simulink library "MESSIN_Library"  (R2024a)
settings: Solver=VariableStepAuto  StartTime=0.0  StopTime=10.0  RelTol=1e-3
undefined symbols (not defined in the file or in its folder): actuatorCommand, commandedActuator, commandMode, externCommand, ready, remoteControlDevice, sensor, supervisor, timestampUTC, useXNAllocation
libraries: $bdroot x376, etargetslib x52, simulink x19
(part 4 of 5)

== system MESSIN_Library/State Message/Unpack MESSIN State Message/unpack message/Unpack AirMAR ==
  busIn : Inport
  bytes : Inport  Port=2
  Bus Assignment : BusAssignment  AssignedSignals=sensor.airMAR.air.timestampUTC,sensor.airMAR.air.pressure,sensor.airMAR.air.airTemperature,sensor.airMAR.relativeWind.timestampUTC,sensor.airMAR.relativeWind.windAngle,sensor.airMAR.relativeWind.windSpeed
  Byte Unpack : etargetslib/Byte Unpack  dimensions={1,1,1,1,1,1}  datatypes={'double','single','single','double','single','single'}  byteAlign=1
      settings: LibrarySourceBlock=embeddedtargetslib/Host Communication/Byte Unpack
  Convert Double Network Byte Order : $bdroot/Utilities/Convert Double Network Byte Order
  Convert Double Network Byte Order1 : $bdroot/Utilities/Convert Double Network Byte Order
  Convert Single Network Byte Order{,1..3} (4 alike) : $bdroot/Utilities/Convert Single Network Byte Order
  Data Type Conversion{1..2,9..12} (6 alike) : DataTypeConversion  OutDataTypeStr=double  SaturateOnIntegerOverflow=off  RndMeth=Floor
  Signal Specification1 : SignalSpecification  OutDataTypeStr=double  Unit=s  Dimensions=1
  Signal Specification12 : SignalSpecification  OutDataTypeStr=double  Unit=s  Dimensions=1
  Signal Specification17 : SignalSpecification  OutDataTypeStr=double  Unit=rad  Dimensions=1
  Signal Specification18 : SignalSpecification  OutDataTypeStr=double  Unit=m/s  Dimensions=1
  Signal Specification2 : SignalSpecification  OutDataTypeStr=double  Unit=Pa  Dimensions=1
  Signal Specification3 : SignalSpecification  OutDataTypeStr=double  Unit=°C  Dimensions=1
  busOut : Outport
  wires:
  Bus Assignment/1 -> busOut/1
  bytes/1 -> Byte Unpack/1
  busIn/1 -> Bus Assignment/1
  Byte Unpack/1 -> Convert Double Network Byte Order/1
  Byte Unpack/2 -> Convert Single Network Byte Order/1
  Byte Unpack/3 -> Convert Single Network Byte Order1/1
  Data Type Conversion9/1 -> Signal Specification1/1
  Data Type Conversion10/1 -> Signal Specification2/1
  Data Type Conversion11/1 -> Signal Specification3/1
  Data Type Conversion12/1 -> Signal Specification12/1
  Data Type Conversion2/1 -> Signal Specification18/1
  Data Type Conversion1/1 -> Signal Specification17/1
  Signal Specification1/1 -> Bus Assignment/2  "timestampUTC"
  Signal Specification12/1 -> Bus Assignment/5  "timestampUTC"
  Signal Specification17/1 -> Bus Assignment/6  "windAngle"
  Signal Specification2/1 -> Bus Assignment/3  "pressure"
  Signal Specification18/1 -> Bus Assignment/7  "windSpeed"
  Signal Specification3/1 -> Bus Assignment/4  "airTemperature"
  Convert Double Network Byte Order/1 -> Data Type Conversion9/1
  Convert Single Network Byte Order/1 -> Data Type Conversion10/1
  Convert Single Network Byte Order1/1 -> Data Type Conversion11/1
  Byte Unpack/4 -> Convert Double Network Byte Order1/1
  Byte Unpack/5 -> Convert Single Network Byte Order2/1
  Byte Unpack/6 -> Convert Single Network Byte Order3/1
  Convert Double Network Byte Order1/1 -> Data Type Conversion12/1
  Convert Single Network Byte Order2/1 -> Data Type Conversion1/1
  Convert Single Network Byte Order3/1 -> Data Type Conversion2/1

== system MESSIN_Library/State Message/Unpack MESSIN State Message/unpack message/Unpack AllocationCommand ==
  busIn : Inport
  bytes : Inport  Port=2
  Bus Assignment : BusAssignment  AssignedSignals=externCommand.allocationCommand.XYN
  Byte Unpack : etargetslib/Byte Unpack  dimensions={1,1,1}  datatypes={'double','double','double'}  byteAlign=1
      settings: LibrarySourceBlock=embeddedtargetslib/Host Communication/Byte Unpack
  Convert Double Network Byte Order : $bdroot/Utilities/Convert Double Network Byte Order
  Convert Double Network Byte Order1 : $bdroot/Utilities/Convert Double Network Byte Order
  Convert Double Network Byte Order2 : $bdroot/Utilities/Convert Double Network Byte Order
  Make Finite : $bdroot/Utilities/Make Finite
  Make Finite1 : $bdroot/Utilities/Make Finite
  Make Finite2 : $bdroot/Utilities/Make Finite
  Mux : Mux  Inputs=3
  Signal Specification1 : SignalSpecification  OutDataTypeStr=double  Dimensions=3
  busOut : Outport
  wires:
  Byte Unpack/3 -> Convert Double Network Byte Order2/1
  Byte Unpack/2 -> Convert Double Network Byte Order1/1
  Byte Unpack/1 -> Convert Double Network Byte Order/1
  Convert Double Network Byte Order2/1 -> Make Finite2/1
  Convert Double Network Byte Order1/1 -> Make Finite1/1
  Convert Double Network Byte Order/1 -> Make Finite/1
  Bus Assignment/1 -> busOut/1
  bytes/1 -> Byte Unpack/1
  busIn/1 -> Bus Assignment/1
  Signal Specification1/1 -> Bus Assignment/2  "XYN"
  Make Finite2/1 -> Mux/3
  Make Finite1/1 -> Mux/2
  Make Finite/1 -> Mux/1
  Mux/1 -> Signal Specification1/1

== system MESSIN_Library/State Message/Unpack MESSIN State Message/unpack message/Unpack BMS ==
  busIn : Inport
  bytes : Inport  Port=2
  Bus Assignment : BusAssignment  AssignedSignals=sensor.batteryManagementSystem.batteryStarboard.timestampUTC,sensor.batteryManagementSystem.batteryStarboard.voltage,sensor.batteryManagementSystem.batteryStarboard.current,sensor.batteryManagementSystem.batteryStarboard.consumedElectricCharge,sensor.batteryManagementSystem.batteryStarboard.stateOfCharge,sensor.batteryManagementSystem.batteryPortside.timestampUTC,sensor.batteryManagementSystem.batteryPortside.voltage,sensor.batteryManagementSystem.batteryPortside.current,sensor.batteryManagementSystem.batteryPortside.consumedElectricCharge,sensor.batteryManagementSystem.batteryPortside.stateOfCharge
  Byte Unpack : etargetslib/Byte Unpack  dimensions={1,1,1,1,1,1,1,1,1,1}  datatypes={'double','single','single','single','single','double','single','single','single','single'}  byteAlign=1
      settings: LibrarySourceBlock=embeddedtargetslib/Host Communication/Byte Unpack
  Convert Double Network Byte Order : $bdroot/Utilities/Convert Double Network Byte Order
  Convert Double Network Byte Order2 : $bdroot/Utilities/Convert Double Network Byte Order
  Convert Single Network Byte Order{,1..7} (8 alike) : $bdroot/Utilities/Convert Single Network Byte Order
  Data Type Conversion{1..3,5..11} (10 alike) : DataTypeConversion  OutDataTypeStr=double  SaturateOnIntegerOverflow=off  RndMeth=Floor
  Signal Specification17 : SignalSpecification  OutDataTypeStr=double  Unit=A*s  Dimensions=1
  Signal Specification18 : SignalSpecification  OutDataTypeStr=double  Unit=1  Dimensions=1
  Signal Specification19 : SignalSpecification  OutDataTypeStr=double  Unit=A*s  Dimensions=1
  Signal Specification20 : SignalSpecification  OutDataTypeStr=double  Unit=1  Dimensions=1
  Signal Specification21 : SignalSpecification  OutDataTypeStr=double  Unit=s  Dimensions=1
  Signal Specification22 : SignalSpecification  OutDataTypeStr=double  Unit=V  Dimensions=1
  Signal Specification23 : SignalSpecification  OutDataTypeStr=double  Unit=A  Dimensions=1
  Signal Specification24 : SignalSpecification  OutDataTypeStr=double  Unit=s  Dimensions=1
  Signal Specification25 : SignalSpecification  OutDataTypeStr=double  Unit=V  Dimensions=1
  Signal Specification26 : SignalSpecification  OutDataTypeStr=double  Unit=A  Dimensions=1
  busOut : Outport
  wires:
  busIn/1 -> Bus Assignment/1
  bytes/1 -> Byte Unpack/1
  Bus Assignment/1 -> busOut/1
  Convert Double Network Byte Order/1 -> Data Type Conversion5/1
  Convert Single Network Byte Order/1 -> Data Type Conversion6/1
  Convert Single Network Byte Order1/1 -> Data Type Conversion7/1
  Convert Single Network Byte Order2/1 -> Data Type Conversion8/1
  Convert Double Network Byte Order2/1 -> Data Type Conversion10/1
  Convert Single Network Byte Order4/1 -> Data Type Conversion11/1
  Convert Single Network Byte Order3/1 -> Data Type Conversion9/1
  Data Type Conversion5/1 -> Signal Specification24/1
  Data Type Conversion6/1 -> Signal Specification25/1
  Data Type Conversion7/1 -> Signal Specification26/1
  Data Type Conversion8/1 -> Signal Specification17/1
  Data Type Conversion9/1 -> Signal Specification18/1
  Data Type Conversion10/1 -> Signal Specification21/1
  Data Type Conversion11/1 -> Signal Specification22/1
  Signal Specification24/1 -> Bus Assignment/2  "timestampUTC"
  Signal Specification19/1 -> Bus Assignment/10  "consumedElectricCharge"
  Signal Specification20/1 -> Bus Assignment/11  "stateOfCharge"
  Signal Specification25/1 -> Bus Assignment/3  "voltage"
  Signal Specification26/1 -> Bus Assignment/4  "current"
  Signal Specification21/1 -> Bus Assignment/7  "timestampUTC"
  Signal Specification17/1 -> Bus Assignment/5  "consumedElectricCharge"
  Signal Specification22/1 -> Bus Assignment/8  "voltage"
  Signal Specification23/1 -> Bus Assignment/9  "current"
  Signal Specification18/1 -> Bus Assignment/6  "stateOfCharge"
  Data Type Conversion2/1 -> Signal Specification20/1
  Data Type Conversion1/1 -> Signal Specification19/1
  Data Type Conversion3/1 -> Signal Specification23/1
  Convert Single Network Byte Order7/1 -> Data Type Conversion3/1
  Convert Single Network Byte Order6/1 -> Data Type Conversion2/1
  Convert Single Network Byte Order5/1 -> Data Type Conversion1/1
  Byte Unpack/1 -> Convert Double Network Byte Order/1
  Byte Unpack/2 -> Convert Single Network Byte Order/1
  Byte Unpack/3 -> Convert Single Network Byte Order1/1
  Byte Unpack/4 -> Convert Single Network Byte Order2/1
  Byte Unpack/5 -> Convert Single Network Byte Order3/1
  Byte Unpack/6 -> Convert Double Network Byte Order2/1
  Byte Unpack/7 -> Convert Single Network Byte Order4/1
  Byte Unpack/8 -> Convert Single Network Byte Order7/1
  Byte Unpack/9 -> Convert Single Network Byte Order5/1
  Byte Unpack/10 -> Convert Single Network Byte Order6/1

== system MESSIN_Library/State Message/Unpack MESSIN State Message/unpack message/Unpack CommandedActuator ==
  busIn : Inport
  bytes : Inport  Port=2
  Bus Assignment : BusAssignment  AssignedSignals=commandedActuator.throttleStarboard,commandedActuator.throttlePortside,commandedActuator.angleStarboard,commandedActuator.anglePortside
  Byte Unpack : etargetslib/Byte Unpack  dimensions={1,1,1,1}  datatypes={'double','double','double','double'}  byteAlign=1
      settings: LibrarySourceBlock=embeddedtargetslib/Host Communication/Byte Unpack
  Convert Double Network Byte Order{,1..3} (4 alike) : $bdroot/Utilities/Convert Double Network Byte Order
  Data Type Conversion{5..8} (4 alike) : DataTypeConversion  OutDataTypeStr=double  SaturateOnIntegerOverflow=off  RndMeth=Floor
  Make Finite{,1..3} (4 alike) : $bdroot/Utilities/Make Finite
  Signal Specification1 : SignalSpecification  OutDataTypeStr=double  Unit=1  Dimensions=1
  Signal Specification2 : SignalSpecification  OutDataTypeStr=double  Unit=1  Dimensions=1
  Signal Specification3 : SignalSpecification  OutDataTypeStr=double  Unit=rad  Dimensions=1
  Signal Specification4 : SignalSpecification  OutDataTypeStr=double  Unit=rad  Dimensions=1
  busOut : Outport
  wires:
  Byte Unpack/4 -> Convert Double Network Byte Order3/1
  Byte Unpack/3 -> Convert Double Network Byte Order2/1
  Byte Unpack/2 -> Convert Double Network Byte Order1/1
  Byte Unpack/1 -> Convert Double Network Byte Order/1
  Make Finite3/1 -> Signal Specification4/1
  Make Finite2/1 -> Signal Specification3/1
  Make Finite1/1 -> Signal Specification1/1
  Data Type Conversion6/1 -> Make Finite1/1
  Make Finite/1 -> Signal Specification2/1
  Convert Double Network Byte Order3/1 -> Data Type Conversion8/1
  Convert Double Network Byte Order2/1 -> Data Type Conversion7/1
  Convert Double Network Byte Order1/1 -> Data Type Conversion6/1
  Convert Double Network Byte Order/1 -> Data Type Conversion5/1
  Data Type Conversion8/1 -> Make Finite3/1
  Data Type Conversion7/1 -> Make Finite2/1
  Data Type Conversion5/1 -> Make Finite/1
  Bus Assignment/1 -> busOut/1
  bytes/1 -> Byte Unpack/1
  busIn/1 -> Bus Assignment/1
  Signal Specification4/1 -> Bus Assignment/5  "anglePortside"
  Signal Specification3/1 -> Bus Assignment/4  "angleStarboard"
  Signal Specification1/1 -> Bus Assignment/3  "throttlePortside"
  Signal Specification2/1 -> Bus Assignment/2  "throttleStarboard"

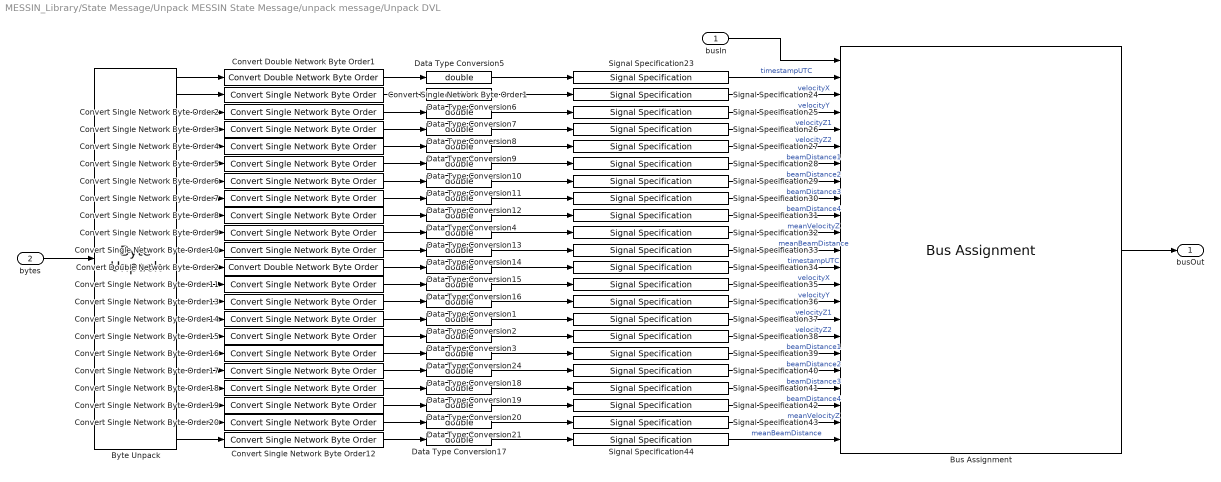
== system MESSIN_Library/State Message/Unpack MESSIN State Message/unpack message/Unpack DVL ==
  busIn : Inport
  bytes : Inport  Port=2
  Bus Assignment : BusAssignment  AssignedSignals=sensor.nortekDVL1000.bottomTrack.timestampUTC,sensor.nortekDVL1000.bottomTrack.velocityX,sensor.nortekDVL1000.bottomTrack.velocityY,sensor.nortekDVL1000.bottomTrack.velocityZ1,sensor.nortekDVL1000.bottomTrack.velocityZ2,sensor.nortekDVL1000.bottomTrack.beamDistance1,sensor.nortekDVL1000.bottomTrack.beamDistance2,sensor.nortekDVL1000.bottomTrack.beamDistance3,sensor.nortekDVL1000.bottomTrack.beamDistance4,sensor.nortekDVL1000.bottomTrack.meanVelocityZ,sensor.nortekDVL1000.bottomTrack.meanBeamDistance,sensor.nortekDVL1000.waterTrack.timestampUTC,sensor.nortekDVL1000.waterTrack.velocityX,sensor.nortekDVL1000.waterTrack.velocityY,sensor.nortekDVL1000.waterTrack.velocityZ1,sensor.nortekDVL1000.waterTrack.velocityZ2,sensor.nortekDVL1000.waterTrack.beamDistance1,sensor.nortekDVL1000.waterTrack.beamDistance2,sensor.nortekDVL1000.waterTrack.beamDistance3,sensor.nortekDVL1000.waterTrack.beamDistance4,sensor.nortekDVL1000.waterTrack.meanVelocityZ,sensor.nortekDVL1000.waterTrack.meanBeamDistance
  Byte Unpack : etargetslib/Byte Unpack  dimensions={1,1,1,1,1,1,1,1,1,1,1,1,1,1,1,1,1,1,1,1,1,1}  datatypes={'double','single','single','single','single','single','single','single','single','single','single','double','single','single','single','single','single','single','single','single','single','single'}  byteAlign=1
      settings: LibrarySourceBlock=embeddedtargetslib/Host Communication/Byte Unpack
  Convert Double Network Byte Order1 : $bdroot/Utilities/Convert Double Network Byte Order
  Convert Double Network Byte Order2 : $bdroot/Utilities/Convert Double Network Byte Order
  Convert Single Network Byte Order{1..20} (20 alike) : $bdroot/Utilities/Convert Single Network Byte Order
  Data Type Conversion{1..21,24} (22 alike) : DataTypeConversion  OutDataTypeStr=double  SaturateOnIntegerOverflow=off  RndMeth=Floor
  Signal Specification23 : SignalSpecification  OutDataTypeStr=double  Unit=s  Dimensions=1
  Signal Specification{24..27,32,35..38,43} (10 alike) : SignalSpecification  OutDataTypeStr=double  Unit=m/s  Dimensions=1
  Signal Specification{28..31,33,39..42,44} (10 alike) : SignalSpecification  OutDataTypeStr=double  Unit=m  Dimensions=1
  Signal Specification34 : SignalSpecification  OutDataTypeStr=double  Unit=s  Dimensions=1
  busOut : Outport
  wires:
  Bus Assignment/1 -> busOut/1
  bytes/1 -> Byte Unpack/1
  busIn/1 -> Bus Assignment/1
  Signal Specification28/1 -> Bus Assignment/7  "beamDistance1"
  Signal Specification31/1 -> Bus Assignment/10  "beamDistance4"
  Signal Specification38/1 -> Bus Assignment/17  "velocityZ2"
  Signal Specification39/1 -> Bus Assignment/18  "beamDistance1"
  Signal Specification30/1 -> Bus Assignment/9  "beamDistance3"
  Signal Specification33/1 -> Bus Assignment/12  "meanBeamDistance"
  Signal Specification41/1 -> Bus Assignment/20  "beamDistance3"
  Signal Specification34/1 -> Bus Assignment/13  "timestampUTC"
  Signal Specification29/1 -> Bus Assignment/8  "beamDistance2"
  Signal Specification42/1 -> Bus Assignment/21  "beamDistance4"
  Signal Specification44/1 -> Bus Assignment/23  "meanBeamDistance"
  Signal Specification25/1 -> Bus Assignment/4  "velocityY"
  Signal Specification26/1 -> Bus Assignment/5  "velocityZ1"
  Signal Specification43/1 -> Bus Assignment/22  "meanVelocityZ"
  Signal Specification36/1 -> Bus Assignment/15  "velocityY"
  Signal Specification32/1 -> Bus Assignment/11  "meanVelocityZ"
  Signal Specification27/1 -> Bus Assignment/6  "velocityZ2"
  Signal Specification23/1 -> Bus Assignment/2  "timestampUTC"
  Signal Specification24/1 -> Bus Assignment/3  "velocityX"
  Signal Specification37/1 -> Bus Assignment/16  "velocityZ1"
  Signal Specification35/1 -> Bus Assignment/14  "velocityX"
  Signal Specification40/1 -> Bus Assignment/19  "beamDistance2"
  Data Type Conversion5/1 -> Signal Specification23/1
  Data Type Conversion6/1 -> Signal Specification24/1
  Data Type Conversion7/1 -> Signal Specification25/1
  Data Type Conversion8/1 -> Signal Specification26/1
  Data Type Conversion9/1 -> Signal Specification27/1
  Data Type Conversion10/1 -> Signal Specification28/1
  Data Type Conversion11/1 -> Signal Specification29/1
  Data Type Conversion12/1 -> Signal Specification30/1
  Data Type Conversion3/1 -> Signal Specification38/1
  Data Type Conversion2/1 -> Signal Specification37/1
  Data Type Conversion1/1 -> Signal Specification36/1
  Data Type Conversion16/1 -> Signal Specification35/1
  Data Type Conversion15/1 -> Signal Specification34/1
  Data Type Conversion14/1 -> Signal Specification33/1
  Data Type Conversion13/1 -> Signal Specification32/1
  Data Type Conversion4/1 -> Signal Specification31/1
  Data Type Conversion24/1 -> Signal Specification39/1
  Data Type Conversion18/1 -> Signal Specification40/1
  Data Type Conversion19/1 -> Signal Specification41/1
  Data Type Conversion20/1 -> Signal Specification42/1
  Data Type Conversion21/1 -> Signal Specification43/1
  Data Type Conversion17/1 -> Signal Specification44/1
  Convert Double Network Byte Order1/1 -> Data Type Conversion5/1
  Convert Single Network Byte Order1/1 -> Data Type Conversion6/1
  Convert Single Network Byte Order2/1 -> Data Type Conversion7/1
  Convert Single Network Byte Order3/1 -> Data Type Conversion8/1
  Convert Single Network Byte Order4/1 -> Data Type Conversion9/1
  Convert Single Network Byte Order5/1 -> Data Type Conversion10/1
  Convert Single Network Byte Order6/1 -> Data Type Conversion11/1
  Convert Single Network Byte Order9/1 -> Data Type Conversion13/1
  Convert Single Network Byte Order8/1 -> Data Type Conversion4/1
  Convert Single Network Byte Order7/1 -> Data Type Conversion12/1
  Convert Single Network Byte Order10/1 -> Data Type Conversion14/1
  Convert Single Network Byte Order12/1 -> Data Type Conversion17/1
  Convert Single Network Byte Order18/1 -> Data Type Conversion19/1
  Convert Single Network Byte Order19/1 -> Data Type Conversion20/1
  Convert Single Network Byte Order20/1 -> Data Type Conversion21/1
  Convert Single Network Byte Order17/1 -> Data Type Conversion18/1
  Convert Single Network Byte Order16/1 -> Data Type Conversion24/1
  Convert Single Network Byte Order15/1 -> Data Type Conversion3/1
  Convert Single Network Byte Order14/1 -> Data Type Conversion2/1
  Convert Single Network Byte Order13/1 -> Data Type Conversion1/1
  Convert Single Network Byte Order11/1 -> Data Type Conversion16/1
  Convert Double Network Byte Order2/1 -> Data Type Conversion15/1
  Byte Unpack/1 -> Convert Double Network Byte Order1/1
  Byte Unpack/2 -> Convert Single Network Byte Order1/1
  Byte Unpack/3 -> Convert Single Network Byte Order2/1
  Byte Unpack/4 -> Convert Single Network Byte Order3/1
  Byte Unpack/5 -> Convert Single Network Byte Order4/1
  Byte Unpack/6 -> Convert Single Network Byte Order5/1
  Byte Unpack/7 -> Convert Single Network Byte Order6/1
  Byte Unpack/8 -> Convert Single Network Byte Order7/1
  Byte Unpack/9 -> Convert Single Network Byte Order8/1
  Byte Unpack/10 -> Convert Single Network Byte Order9/1
  Byte Unpack/11 -> Convert Single Network Byte Order10/1
  Byte Unpack/12 -> Convert Double Network Byte Order2/1
  Byte Unpack/13 -> Convert Single Network Byte Order11/1
  Byte Unpack/14 -> Convert Single Network Byte Order13/1
  Byte Unpack/15 -> Convert Single Network Byte Order14/1
  Byte Unpack/16 -> Convert Single Network Byte Order15/1
  Byte Unpack/17 -> Convert Single Network Byte Order16/1
  Byte Unpack/18 -> Convert Single Network Byte Order17/1
  Byte Unpack/19 -> Convert Single Network Byte Order18/1
  Byte Unpack/20 -> Convert Single Network Byte Order19/1
  Byte Unpack/21 -> Convert Single Network Byte Order20/1
  Byte Unpack/22 -> Convert Single Network Byte Order12/1

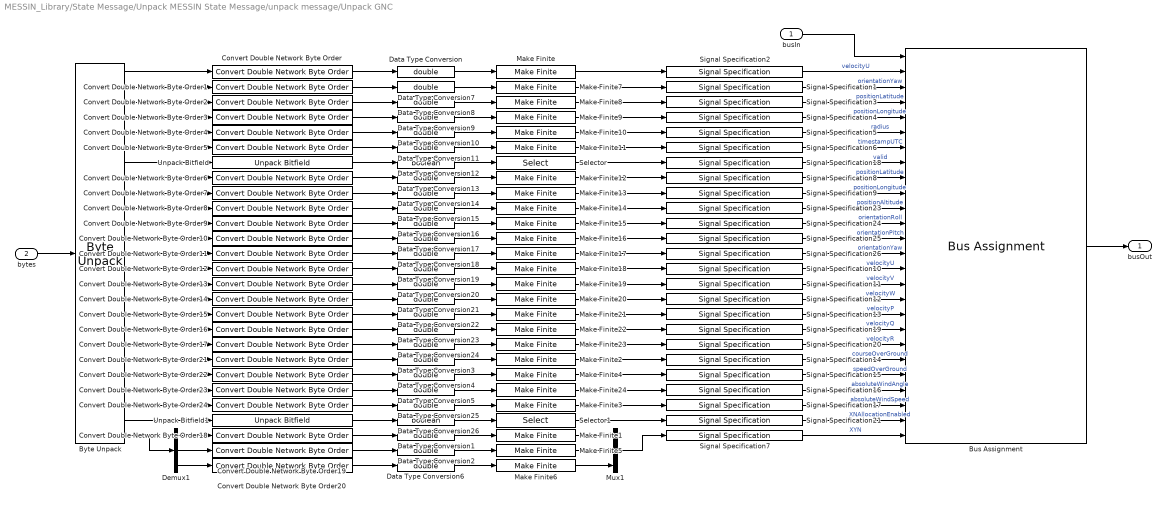
== system MESSIN_Library/State Message/Unpack MESSIN State Message/unpack message/Unpack GNC ==
  busIn : Inport
  bytes : Inport  Port=2
  Bus Assignment : BusAssignment  AssignedSignals=gnc.guidance.surgeHeading.velocityU,gnc.guidance.surgeHeading.orientationYaw,gnc.guidance.stayThere.positionLatitude,gnc.guidance.stayThere.positionLongitude,gnc.guidance.stayThere.radius,gnc.navigation.timestampUTC,gnc.navigation.info.valid,gnc.navigation.state.positionLatitude,gnc.navigation.state.positionLongitude,gnc.navigation.state.positionAltitude,gnc.navigation.state.orientationRoll,gnc.navigation.state.orientationPitch,gnc.navigation.state.orientationYaw,gnc.navigation.state.velocityU,gnc.navigation.state.velocityV,gnc.navigation.state.velocityW,gnc.navigation.state.velocityP,gnc.navigation.state.velocityQ,gnc.navigation.state.velocityR,gnc.navigation.state.courseOverGround,gnc.navigation.state.speedOverGround,gnc.navigation.state.absoluteWindAngle,gnc.navigation.state.absoluteWindSpeed,gnc.control.XNAllocationEnabled,gnc.control.XYN
  Byte Unpack : etargetslib/Byte Unpack  dimensions={1,1,1,1,1,1,1,1,1,1,1,1,1,1,1,1,1,1,1,1,1,1,1,1,3}  datatypes={'double','double','double','double','double','double','uint8','double','double','double','double','double','double','double','double','double','double','double','double','double','double','double','double','uint8','double'}  byteAlign=1
      settings: LibrarySourceBlock=embeddedtargetslib/Host Communication/Byte Unpack
  Convert Double Network Byte Order{,1..24} (25 alike) : $bdroot/Utilities/Convert Double Network Byte Order
  Data Type Conversion{,1..11,13..25} (25 alike) : DataTypeConversion  OutDataTypeStr=double  SaturateOnIntegerOverflow=off  RndMeth=Floor
  Data Type Conversion12 : DataTypeConversion  OutDataTypeStr=boolean  SaturateOnIntegerOverflow=off  RndMeth=Floor
  Data Type Conversion26 : DataTypeConversion  OutDataTypeStr=boolean  SaturateOnIntegerOverflow=off  RndMeth=Floor
  Demux1 : Demux  Outputs=3
  Make Finite{,1..24} (25 alike) : $bdroot/Utilities/Make Finite
  Mux1 : Mux  Inputs=3
  Selector : Selector  InputPortWidth=8  IndexOptions=Index vector (dialog)  Indices=8  OutputSizes=1
  Selector1 : Selector  InputPortWidth=8  IndexOptions=Index vector (dialog)  Indices=8  OutputSizes=1
  Signal Specification{1,3..4,8..9,14,16,24..26} (10 alike) : SignalSpecification  OutDataTypeStr=double  Unit=rad  Dimensions=1
  Signal Specification{2,10..12,15,17} (6 alike) : SignalSpecification  OutDataTypeStr=double  Unit=m/s  Dimensions=1
  Signal Specification13 : SignalSpecification  OutDataTypeStr=double  Unit=rad/s  Dimensions=1
  Signal Specification18 : SignalSpecification  OutDataTypeStr=boolean  Unit=1  Dimensions=1
  Signal Specification19 : SignalSpecification  OutDataTypeStr=double  Unit=rad/s  Dimensions=1
  Signal Specification20 : SignalSpecification  OutDataTypeStr=double  Unit=rad/s  Dimensions=1
  Signal Specification21 : SignalSpecification  OutDataTypeStr=boolean  Unit=1  Dimensions=1
  Signal Specification23 : SignalSpecification  OutDataTypeStr=double  Unit=m  Dimensions=1
  Signal Specification5 : SignalSpecification  OutDataTypeStr=double  Unit=m  Dimensions=1
  Signal Specification6 : SignalSpecification  OutDataTypeStr=double  Unit=s  Dimensions=1
  Signal Specification7 : SignalSpecification  OutDataTypeStr=double  Dimensions=3
  Unpack Bitfield : $bdroot/Utilities/Unpack Bitfield
  Unpack Bitfield1 : $bdroot/Utilities/Unpack Bitfield
  busOut : Outport
  wires:
  Data Type Conversion6/1 -> Make Finite6/1
  Data Type Conversion2/1 -> Make Finite5/1
  Data Type Conversion1/1 -> Make Finite1/1
  Convert Double Network Byte Order18/1 -> Data Type Conversion1/1
  Convert Double Network Byte Order19/1 -> Data Type Conversion2/1
  Convert Double Network Byte Order20/1 -> Data Type Conversion6/1
  Make Finite6/1 -> Mux1/3
  Make Finite5/1 -> Mux1/2
  Make Finite1/1 -> Mux1/1
  Demux1/1 -> Convert Double Network Byte Order18/1
  Demux1/2 -> Convert Double Network Byte Order19/1
  Demux1/3 -> Convert Double Network Byte Order20/1
  Convert Double Network Byte Order/1 -> Data Type Conversion/1
  Data Type Conversion/1 -> Make Finite/1
  busIn/1 -> Bus Assignment/1
  bytes/1 -> Byte Unpack/1
  Bus Assignment/1 -> busOut/1
  Signal Specification3/1 -> Bus Assignment/4  "positionLatitude"
  Signal Specification2/1 -> Bus Assignment/2  "velocityU"
  Signal Specification4/1 -> Bus Assignment/5  "positionLongitude"
  Signal Specification1/1 -> Bus Assignment/3  "orientationYaw"
  Signal Specification5/1 -> Bus Assignment/6  "radius"
  Signal Specification25/1 -> Bus Assignment/13  "orientationPitch"
  Signal Specification23/1 -> Bus Assignment/11  "positionAltitude"
  Signal Specification20/1 -> Bus Assignment/20  "velocityR"
  Signal Specification8/1 -> Bus Assignment/9  "positionLatitude"
  Signal Specification10/1 -> Bus Assignment/15  "velocityU"
  Signal Specification13/1 -> Bus Assignment/18  "velocityP"
  Signal Specification19/1 -> Bus Assignment/19  "velocityQ"
  Signal Specification18/1 -> Bus Assignment/8  "valid"
  Signal Specification11/1 -> Bus Assignment/16  "velocityV"
  Signal Specification6/1 -> Bus Assignment/7  "timestampUTC"
  Signal Specification12/1 -> Bus Assignment/17  "velocityW"
  Signal Specification26/1 -> Bus Assignment/14  "orientationYaw"
  Signal Specification9/1 -> Bus Assignment/10  "positionLongitude"
  Signal Specification24/1 -> Bus Assignment/12  "orientationRoll"
  Signal Specification7/1 -> Bus Assignment/26  "XYN"
  Make Finite/1 -> Signal Specification2/1
  Make Finite7/1 -> Signal Specification1/1
  Data Type Conversion7/1 -> Make Finite7/1
  Convert Double Network Byte Order1/1 -> Data Type Conversion7/1
  Convert Double Network Byte Order3/1 -> Data Type Conversion9/1
  Data Type Conversion9/1 -> Make Finite9/1
  Make Finite9/1 -> Signal Specification4/1
  Make Finite8/1 -> Signal Specification3/1
  Data Type Conversion8/1 -> Make Finite8/1
  Convert Double Network Byte Order2/1 -> Data Type Conversion8/1
  Convert Double Network Byte Order4/1 -> Data Type Conversion10/1
  Data Type Conversion10/1 -> Make Finite10/1
  Make Finite10/1 -> Signal Specification5/1
  Make Finite11/1 -> Signal Specification6/1
  Data Type Conversion11/1 -> Make Finite11/1
  Convert Double Network Byte Order5/1 -> Data Type Conversion11/1
  Data Type Conversion12/1 -> Selector/1
  Unpack Bitfield/1 -> Data Type Conversion12/1
  Selector/1 -> Signal Specification18/1
  Convert Double Network Byte Order8/1 -> Data Type Conversion15/1
  Data Type Conversion15/1 -> Make Finite14/1
  Make Finite14/1 -> Signal Specification23/1
  Make Finite15/1 -> Signal Specification24/1
  Data Type Conversion16/1 -> Make Finite15/1
  Convert Double Network Byte Order9/1 -> Data Type Conversion16/1
  Convert Double Network Byte Order7/1 -> Data Type Conversion14/1
  Data Type Conversion14/1 -> Make Finite13/1
  Make Finite13/1 -> Signal Specification9/1
  Make Finite12/1 -> Signal Specification8/1
  Data Type Conversion13/1 -> Make Finite12/1
  Convert Double Network Byte Order6/1 -> Data Type Conversion13/1
  Convert Double Network Byte Order10/1 -> Data Type Conversion17/1
  Data Type Conversion17/1 -> Make Finite16/1
  Make Finite16/1 -> Signal Specification25/1
  Make Finite17/1 -> Signal Specification26/1
  Data Type Conversion18/1 -> Make Finite17/1
  Convert Double Network Byte Order11/1 -> Data Type Conversion18/1
  Convert Double Network Byte Order13/1 -> Data Type Conversion20/1
  Data Type Conversion20/1 -> Make Finite19/1
  Make Finite19/1 -> Signal Specification11/1
  Make Finite18/1 -> Signal Specification10/1
  Data Type Conversion19/1 -> Make Finite18/1
  Convert Double Network Byte Order12/1 -> Data Type Conversion19/1
  Convert Double Network Byte Order16/1 -> Data Type Conversion23/1
  Data Type Conversion23/1 -> Make Finite22/1
  Make Finite22/1 -> Signal Specification19/1
  Make Finite23/1 -> Signal Specification20/1
  Data Type Conversion24/1 -> Make Finite23/1
  Convert Double Network Byte Order17/1 -> Data Type Conversion24/1
  Convert Double Network Byte Order15/1 -> Data Type Conversion22/1
  Data Type Conversion22/1 -> Make Finite21/1
  Make Finite21/1 -> Signal Specification13/1
  Make Finite20/1 -> Signal Specification12/1
  Data Type Conversion21/1 -> Make Finite20/1
  Convert Double Network Byte Order14/1 -> Data Type Conversion21/1
  Mux1/1 -> Signal Specification7/1
  Byte Unpack/1 -> Convert Double Network Byte Order/1
  Byte Unpack/2 -> Convert Double Network Byte Order1/1
  Byte Unpack/3 -> Convert Double Network Byte Order2/1
  Byte Unpack/4 -> Convert Double Network Byte Order3/1
  Byte Unpack/5 -> Convert Double Network Byte Order4/1
  Byte Unpack/6 -> Convert Double Network Byte Order5/1
  Byte Unpack/7 -> Unpack Bitfield/1
  Byte Unpack/8 -> Convert Double Network Byte Order6/1
  Byte Unpack/9 -> Convert Double Network Byte Order7/1
  Byte Unpack/10 -> Convert Double Network Byte Order8/1
  Byte Unpack/11 -> Convert Double Network Byte Order9/1
  Byte Unpack/12 -> Convert Double Network Byte Order10/1
  Byte Unpack/13 -> Convert Double Network Byte Order11/1
  Byte Unpack/14 -> Convert Double Network Byte Order12/1
  Byte Unpack/15 -> Convert Double Network Byte Order13/1
  Byte Unpack/16 -> Convert Double Network Byte Order14/1
  Byte Unpack/17 -> Convert Double Network Byte Order15/1
  Byte Unpack/18 -> Convert Double Network Byte Order16/1
  Byte Unpack/19 -> Convert Double Network Byte Order17/1
  Convert Double Network Byte Order21/1 -> Data Type Conversion3/1
  Data Type Conversion3/1 -> Make Finite2/1
  Data Type Conversion25/1 -> Make Finite3/1
  Convert Double Network Byte Order24/1 -> Data Type Conversion25/1
  Convert Double Network Byte Order23/1 -> Data Type Conversion5/1
  Data Type Conversion5/1 -> Make Finite24/1
  Data Type Conversion4/1 -> Make Finite4/1
  Convert Double Network Byte Order22/1 -> Data Type Conversion4/1
  Make Finite2/1 -> Signal Specification14/1
  Signal Specification14/1 -> Bus Assignment/21  "courseOverGround"
  Make Finite4/1 -> Signal Specification15/1
  Signal Specification15/1 -> Bus Assignment/22  "speedOverGround"
  Make Finite24/1 -> Signal Specification16/1
  Make Finite3/1 -> Signal Specification17/1
  Signal Specification16/1 -> Bus Assignment/23  "absoluteWindAngle"
  Signal Specification17/1 -> Bus Assignment/24  "absoluteWindSpeed"
  Byte Unpack/20 -> Convert Double Network Byte Order21/1
  Byte Unpack/21 -> Convert Double Network Byte Order22/1
  Byte Unpack/22 -> Convert Double Network Byte Order23/1
  Byte Unpack/23 -> Convert Double Network Byte Order24/1
  Byte Unpack/24 -> Unpack Bitfield1/1
  Unpack Bitfield1/1 -> Data Type Conversion26/1
  Data Type Conversion26/1 -> Selector1/1
  Selector1/1 -> Signal Specification21/1
  Signal Specification21/1 -> Bus Assignment/25  "XNAllocationEnabled"
  Byte Unpack/25 -> Demux1/1

== system MESSIN_Library/State Message/Unpack MESSIN State Message/unpack message/Unpack GNSS ==
  busIn : Inport
  bytes : Inport  Port=2
  Bus Assignment : BusAssignment  AssignedSignals=sensor.gnssAsteRx3.gnss.timestampUTC,sensor.gnssAsteRx3.gnss.latitude,sensor.gnssAsteRx3.gnss.longitude,sensor.gnssAsteRx3.gnss.altitude,sensor.gnssAsteRx3.gnss.hdop,sensor.gnssAsteRx3.gnss.numSat,sensor.gnssAsteRx3.gnss.gpsQuality,sensor.gnssAsteRx3.courseAndSpeedOverGround.timestampUTC,sensor.gnssAsteRx3.courseAndSpeedOverGround.courseOverGround,sensor.gnssAsteRx3.courseAndSpeedOverGround.speedOverGround
  Byte Unpack : etargetslib/Byte Unpack  dimensions={1,1,1,1,1,1,1,1,1,1}  datatypes={'double','double','double','single','single','uint8','uint8','double','single','single'}  byteAlign=1
      settings: LibrarySourceBlock=embeddedtargetslib/Host Communication/Byte Unpack
  Convert Double Network Byte Order{5..8} (4 alike) : $bdroot/Utilities/Convert Double Network Byte Order
  Convert Single Network Byte Order{8..11} (4 alike) : $bdroot/Utilities/Convert Single Network Byte Order
  Data Type Conversion{17,20..21,23..27} (8 alike) : DataTypeConversion  OutDataTypeStr=double  SaturateOnIntegerOverflow=off  RndMeth=Floor
  Data Type Conversion18 : DataTypeConversion  OutDataTypeStr=uint8  SaturateOnIntegerOverflow=off  RndMeth=Floor
  Data Type Conversion19 : DataTypeConversion  OutDataTypeStr=uint8  SaturateOnIntegerOverflow=off  RndMeth=Floor
  Signal Specification45 : SignalSpecification  OutDataTypeStr=double  Unit=m  Dimensions=1
  Signal Specification46 : SignalSpecification  OutDataTypeStr=uint8  Unit=1  Dimensions=1
  Signal Specification47 : SignalSpecification  OutDataTypeStr=double  Unit=m  Dimensions=1
  Signal Specification50 : SignalSpecification  OutDataTypeStr=uint8  Unit=1  Dimensions=1
  Signal Specification51 : SignalSpecification  OutDataTypeStr=double  Unit=s  Dimensions=1
  Signal Specification52 : SignalSpecification  OutDataTypeStr=double  Unit=rad  Dimensions=1
  Signal Specification53 : SignalSpecification  OutDataTypeStr=double  Unit=m/s  Dimensions=1
  Signal Specification54 : SignalSpecification  OutDataTypeStr=double  Unit=s  Dimensions=1
  Signal Specification55 : SignalSpecification  OutDataTypeStr=double  Unit=rad  Dimensions=1
  Signal Specification56 : SignalSpecification  OutDataTypeStr=double  Unit=rad  Dimensions=1
  busOut : Outport
  wires:
  Bus Assignment/1 -> busOut/1
  bytes/1 -> Byte Unpack/1
  busIn/1 -> Bus Assignment/1
  Signal Specification53/1 -> Bus Assignment/11  "speedOverGround"
  Signal Specification46/1 -> Bus Assignment/7  "numSat"
  Signal Specification50/1 -> Bus Assignment/8  "gpsQuality"
  Signal Specification47/1 -> Bus Assignment/6  "hdop"
  Signal Specification55/1 -> Bus Assignment/3  "latitude"
  Signal Specification54/1 -> Bus Assignment/2  "timestampUTC"
  Signal Specification45/1 -> Bus Assignment/5  "altitude"
  Signal Specification52/1 -> Bus Assignment/10  "courseOverGround"
  Signal Specification51/1 -> Bus Assignment/9  "timestampUTC"
  Signal Specification56/1 -> Bus Assignment/4  "longitude"
  Data Type Conversion23/1 -> Signal Specification54/1
  Data Type Conversion24/1 -> Signal Specification55/1
  Data Type Conversion25/1 -> Signal Specification56/1
  Data Type Conversion26/1 -> Signal Specification45/1
  Data Type Conversion27/1 -> Signal Specification47/1
  Data Type Conversion20/1 -> Signal Specification51/1
  Data Type Conversion17/1 -> Signal Specification52/1
  Data Type Conversion21/1 -> Signal Specification53/1
  Data Type Conversion18/1 -> Signal Specification46/1
  Data Type Conversion19/1 -> Signal Specification50/1
  Convert Double Network Byte Order5/1 -> Data Type Conversion23/1
  Convert Double Network Byte Order6/1 -> Data Type Conversion24/1
  Convert Double Network Byte Order7/1 -> Data Type Conversion25/1
  Convert Single Network Byte Order8/1 -> Data Type Conversion26/1
  Convert Single Network Byte Order9/1 -> Data Type Conversion27/1
  Convert Double Network Byte Order8/1 -> Data Type Conversion20/1
  Convert Single Network Byte Order10/1 -> Data Type Conversion17/1
  Convert Single Network Byte Order11/1 -> Data Type Conversion21/1
  Byte Unpack/1 -> Convert Double Network Byte Order5/1
  Byte Unpack/2 -> Convert Double Network Byte Order6/1
  Byte Unpack/3 -> Convert Double Network Byte Order7/1
  Byte Unpack/4 -> Convert Single Network Byte Order8/1
  Byte Unpack/5 -> Convert Single Network Byte Order9/1
  Byte Unpack/6 -> Data Type Conversion18/1
  Byte Unpack/7 -> Data Type Conversion19/1
  Byte Unpack/8 -> Convert Double Network Byte Order8/1
  Byte Unpack/9 -> Convert Single Network Byte Order10/1
  Byte Unpack/10 -> Convert Single Network Byte Order11/1

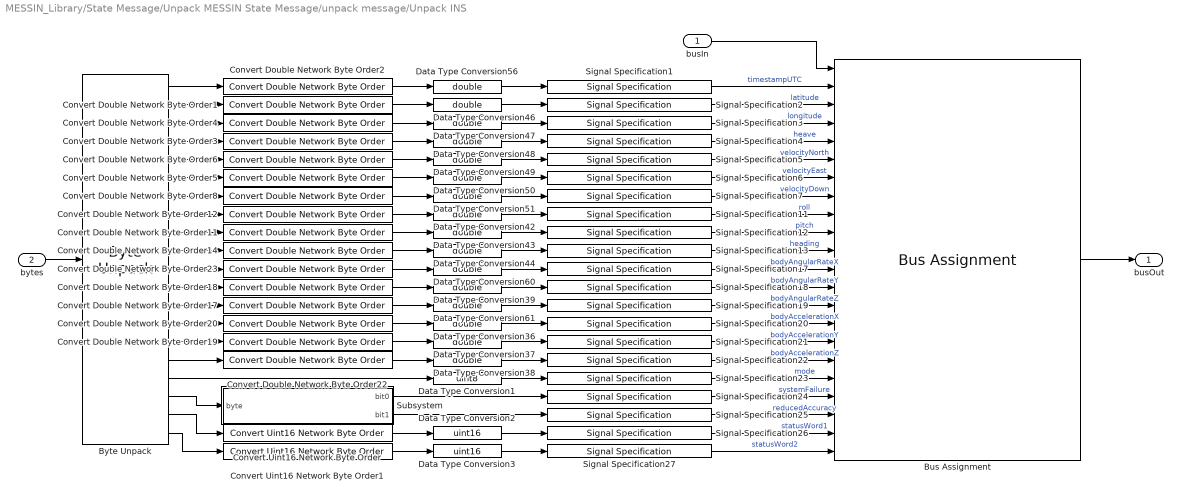
== system MESSIN_Library/State Message/Unpack MESSIN State Message/unpack message/Unpack INS ==
  busIn : Inport
  bytes : Inport  Port=2
  Bus Assignment : BusAssignment  AssignedSignals=sensor.insLFK100.timestampUTC,sensor.insLFK100.latitude,sensor.insLFK100.longitude,sensor.insLFK100.heave,sensor.insLFK100.velocityNorth,sensor.insLFK100.velocityEast,sensor.insLFK100.velocityDown,sensor.insLFK100.roll,sensor.insLFK100.pitch,sensor.insLFK100.heading,sensor.insLFK100.bodyAngularRateX,sensor.insLFK100.bodyAngularRateY,sensor.insLFK100.bodyAngularRateZ,sensor.insLFK100.bodyAccelerationX,sensor.insLFK100.bodyAccelerationY,sensor.insLFK100.bodyAccelerationZ,sensor.insLFK100.details.mode,sensor.insLFK100.details.systemFailure,sensor.insLFK100.details.reducedAccuracy,sensor.insLFK100.details.statusWord1,sensor.insLFK100.details.statusWord2
  Byte Unpack : etargetslib/Byte Unpack  dimensions={1,1,1,1,1,1,1,1,1,1,1,1,1,1,1,1,1,1,1,1}  datatypes={'double','double','double','double','double','double','double','double','double','double','double','double','double','double','double','double','uint8','uint8','uint16','uint16'}  byteAlign=1
      settings: LibrarySourceBlock=embeddedtargetslib/Host Communication/Byte Unpack
  Convert Double Network Byte Order{1..6,8,11..12,14,17..20,22..23} (16 alike) : $bdroot/Utilities/Convert Double Network Byte Order
  Convert Uint16 Network Byte Order : $bdroot/Utilities/Convert Uint16 Network Byte Order
  Convert Uint16 Network Byte Order1 : $bdroot/Utilities/Convert Uint16 Network Byte Order
  Data Type Conversion1 : DataTypeConversion  OutDataTypeStr=uint8  SaturateOnIntegerOverflow=off  RndMeth=Floor
  Data Type Conversion2 : DataTypeConversion  OutDataTypeStr=uint16  SaturateOnIntegerOverflow=off  RndMeth=Floor
  Data Type Conversion3 : DataTypeConversion  OutDataTypeStr=uint16  SaturateOnIntegerOverflow=off  RndMeth=Floor
  Data Type Conversion{36..39,42..44,46..51,56,60..61} (16 alike) : DataTypeConversion  OutDataTypeStr=double  SaturateOnIntegerOverflow=off  RndMeth=Floor
  Signal Specification1 : SignalSpecification  OutDataTypeStr=double  Unit=s  Dimensions=1
  Signal Specification{2..3,11..13} (5 alike) : SignalSpecification  OutDataTypeStr=double  Unit=rad  Dimensions=1
  Signal Specification17 : SignalSpecification  OutDataTypeStr=double  Unit=rad/s  Dimensions=1
  Signal Specification18 : SignalSpecification  OutDataTypeStr=double  Unit=rad/s  Dimensions=1
  Signal Specification19 : SignalSpecification  OutDataTypeStr=double  Unit=rad/s  Dimensions=1
  Signal Specification20 : SignalSpecification  OutDataTypeStr=double  Unit=m/s^2  Dimensions=1
  Signal Specification21 : SignalSpecification  OutDataTypeStr=double  Unit=m/s^2  Dimensions=1
  Signal Specification22 : SignalSpecification  OutDataTypeStr=double  Unit=m/s^2  Dimensions=1
  Signal Specification23 : SignalSpecification  OutDataTypeStr=uint8  Dimensions=1
  Signal Specification24 : SignalSpecification  OutDataTypeStr=boolean  Dimensions=1
  Signal Specification25 : SignalSpecification  OutDataTypeStr=boolean  Dimensions=1
  Signal Specification26 : SignalSpecification  OutDataTypeStr=uint16  Dimensions=1
  Signal Specification27 : SignalSpecification  OutDataTypeStr=uint16  Dimensions=1
  Signal Specification4 : SignalSpecification  OutDataTypeStr=double  Unit=m  Dimensions=1
  Signal Specification5 : SignalSpecification  OutDataTypeStr=double  Unit=m/s  Dimensions=1
  Signal Specification6 : SignalSpecification  OutDataTypeStr=double  Unit=m/s  Dimensions=1
  Signal Specification7 : SignalSpecification  OutDataTypeStr=double  Unit=m/s  Dimensions=1
  Subsystem : Subsystem
  busOut : Outport
  wires:
  Convert Double Network Byte Order17/1 -> Data Type Conversion61/1
  Convert Double Network Byte Order23/1 -> Data Type Conversion60/1
  Convert Double Network Byte Order2/1 -> Data Type Conversion56/1
  Convert Double Network Byte Order1/1 -> Data Type Conversion46/1
  Convert Double Network Byte Order8/1 -> Data Type Conversion51/1
  Convert Double Network Byte Order5/1 -> Data Type Conversion50/1
  Convert Double Network Byte Order6/1 -> Data Type Conversion49/1
  Convert Double Network Byte Order3/1 -> Data Type Conversion48/1
  Convert Double Network Byte Order4/1 -> Data Type Conversion47/1
  Convert Double Network Byte Order12/1 -> Data Type Conversion42/1
  Convert Double Network Byte Order11/1 -> Data Type Conversion43/1
  Convert Double Network Byte Order14/1 -> Data Type Conversion44/1
  Convert Double Network Byte Order18/1 -> Data Type Conversion39/1
  Convert Double Network Byte Order20/1 -> Data Type Conversion36/1
  Convert Double Network Byte Order22/1 -> Data Type Conversion38/1
  Convert Double Network Byte Order19/1 -> Data Type Conversion37/1
  busIn/1 -> Bus Assignment/1
  bytes/1 -> Byte Unpack/1
  Bus Assignment/1 -> busOut/1
  Data Type Conversion47/1 -> Signal Specification3/1
  Data Type Conversion48/1 -> Signal Specification4/1
  Data Type Conversion51/1 -> Signal Specification7/1
  Data Type Conversion50/1 -> Signal Specification6/1
  Data Type Conversion49/1 -> Signal Specification5/1
  Data Type Conversion43/1 -> Signal Specification12/1
  Data Type Conversion44/1 -> Signal Specification13/1
  Data Type Conversion42/1 -> Signal Specification11/1
  Data Type Conversion60/1 -> Signal Specification17/1
  Data Type Conversion61/1 -> Signal Specification19/1
  Data Type Conversion36/1 -> Signal Specification20/1
  Data Type Conversion39/1 -> Signal Specification18/1
  Data Type Conversion37/1 -> Signal Specification21/1
  Data Type Conversion38/1 -> Signal Specification22/1
  Signal Specification1/1 -> Bus Assignment/2  "timestampUTC"
  Signal Specification2/1 -> Bus Assignment/3  "latitude"
  Signal Specification3/1 -> Bus Assignment/4  "longitude"
  Signal Specification4/1 -> Bus Assignment/5  "heave"
  Signal Specification5/1 -> Bus Assignment/6  "velocityNorth"
  Signal Specification6/1 -> Bus Assignment/7  "velocityEast"
  Signal Specification7/1 -> Bus Assignment/8  "velocityDown"
  Signal Specification11/1 -> Bus Assignment/9  "roll"
  Signal Specification12/1 -> Bus Assignment/10  "pitch"
  Signal Specification13/1 -> Bus Assignment/11  "heading"
  Signal Specification17/1 -> Bus Assignment/12  "bodyAngularRateX"
  Signal Specification18/1 -> Bus Assignment/13  "bodyAngularRateY"
  Signal Specification19/1 -> Bus Assignment/14  "bodyAngularRateZ"
  Signal Specification20/1 -> Bus Assignment/15  "bodyAccelerationX"
  Signal Specification21/1 -> Bus Assignment/16  "bodyAccelerationY"
  Signal Specification22/1 -> Bus Assignment/17  "bodyAccelerationZ"
  Signal Specification26/1 -> Bus Assignment/21  "statusWord1"
  Signal Specification25/1 -> Bus Assignment/20  "reducedAccuracy"
  Data Type Conversion2/1 -> Signal Specification26/1
  Subsystem/2(bit1) -> Signal Specification25/1
  Signal Specification27/1 -> Bus Assignment/22  "statusWord2"
  Data Type Conversion1/1 -> Signal Specification23/1
  Signal Specification24/1 -> Bus Assignment/19  "systemFailure"
  Signal Specification23/1 -> Bus Assignment/18  "mode"
  Data Type Conversion3/1 -> Signal Specification27/1
  Subsystem/1(bit0) -> Signal Specification24/1
  Convert Uint16 Network Byte Order/1 -> Data Type Conversion2/1
  Convert Uint16 Network Byte Order1/1 -> Data Type Conversion3/1
  Byte Unpack/16 -> Convert Double Network Byte Order22/1
  Byte Unpack/15 -> Convert Double Network Byte Order19/1
  Byte Unpack/14 -> Convert Double Network Byte Order20/1
  Byte Unpack/13 -> Convert Double Network Byte Order17/1
  Byte Unpack/12 -> Convert Double Network Byte Order18/1
  Byte Unpack/11 -> Convert Double Network Byte Order23/1
  Byte Unpack/10 -> Convert Double Network Byte Order14/1
  Byte Unpack/9 -> Convert Double Network Byte Order11/1
  Byte Unpack/8 -> Convert Double Network Byte Order12/1
  Byte Unpack/7 -> Convert Double Network Byte Order8/1
  Byte Unpack/6 -> Convert Double Network Byte Order5/1
  Byte Unpack/5 -> Convert Double Network Byte Order6/1
  Byte Unpack/4 -> Convert Double Network Byte Order3/1
  Byte Unpack/3 -> Convert Double Network Byte Order4/1
  Byte Unpack/2 -> Convert Double Network Byte Order1/1
  Byte Unpack/1 -> Convert Double Network Byte Order2/1
  Byte Unpack/17 -> Data Type Conversion1/1
  Byte Unpack/18 -> Subsystem/1(byte)
  Byte Unpack/19 -> Convert Uint16 Network Byte Order/1
  Byte Unpack/20 -> Convert Uint16 Network Byte Order1/1
  Data Type Conversion56/1 -> Signal Specification1/1
  Data Type Conversion46/1 -> Signal Specification2/1

== system MESSIN_Library/State Message/Unpack MESSIN State Message/unpack message/Unpack Info ==
  busIn : Inport
  bytes : Inport  Port=2
  Bus Assignment : BusAssignment  AssignedSignals=timestampUTC
  Byte Unpack : etargetslib/Byte Unpack  dimensions={1}  datatypes={'double'}  byteAlign=1
      settings: LibrarySourceBlock=embeddedtargetslib/Host Communication/Byte Unpack
  Convert Double Network Byte Order : $bdroot/Utilities/Convert Double Network Byte Order
  Data Type Conversion : DataTypeConversion  OutDataTypeStr=double  SaturateOnIntegerOverflow=off  RndMeth=Floor
  Make Finite : $bdroot/Utilities/Make Finite
  Signal Specification : SignalSpecification  OutDataTypeStr=double  Unit=s  Dimensions=1
  busOut : Outport
  wires:
  Bus Assignment/1 -> busOut/1
  bytes/1 -> Byte Unpack/1
  busIn/1 -> Bus Assignment/1
  Signal Specification/1 -> Bus Assignment/2
  Convert Double Network Byte Order/1 -> Data Type Conversion/1
  Byte Unpack/1 -> Convert Double Network Byte Order/1
  Data Type Conversion/1 -> Make Finite/1
  Make Finite/1 -> Signal Specification/1

== system MESSIN_Library/State Message/Unpack MESSIN State Message/unpack message/Unpack Info1 ==
  busIn : Inport
  bytes : Inport  Port=2
  Bus Assignment : BusAssignment  AssignedSignals=externCommand.timestampUTC,externCommand.ready,externCommand.useXNAllocation,externCommand.commandMode
  Byte Unpack : etargetslib/Byte Unpack  dimensions={1,1,1}  datatypes={'double','uint8','uint8'}  byteAlign=1
      settings: LibrarySourceBlock=embeddedtargetslib/Host Communication/Byte Unpack
  Convert Double Network Byte Order : $bdroot/Utilities/Convert Double Network Byte Order
  Data Type Conversion : DataTypeConversion  OutDataTypeStr=double  SaturateOnIntegerOverflow=off  RndMeth=Floor
  Data Type Conversion1 : DataTypeConversion  OutDataTypeStr=boolean  SaturateOnIntegerOverflow=off  RndMeth=Floor
  Make Finite : $bdroot/Utilities/Make Finite
  Selector : Selector  InputPortWidth=8  IndexOptions=Index vector (dialog)  Indices=8  OutputSizes=1
  Selector1 : Selector  InputPortWidth=8  IndexOptions=Index vector (dialog)  Indices=7  OutputSizes=1
  Signal Specification : SignalSpecification  OutDataTypeStr=double  Unit=s  Dimensions=1
  Signal Specification1 : SignalSpecification  OutDataTypeStr=boolean  Dimensions=1
  Signal Specification2 : SignalSpecification  OutDataTypeStr=boolean  Dimensions=1
  Unpack Bitfield : $bdroot/Utilities/Unpack Bitfield
  busOut : Outport
  wires:
  Bus Assignment/1 -> busOut/1
  bytes/1 -> Byte Unpack/1
  Byte Unpack/1 -> Convert Double Network Byte Order/1
  Convert Double Network Byte Order/1 -> Data Type Conversion/1
  busIn/1 -> Bus Assignment/1
  Signal Specification/1 -> Bus Assignment/2
  Data Type Conversion/1 -> Make Finite/1
  Make Finite/1 -> Signal Specification/1
  Byte Unpack/2 -> Unpack Bitfield/1
  Unpack Bitfield/1 -> Data Type Conversion1/1
  Data Type Conversion1/1 -> Selector1/1, Selector/1
  Selector/1 -> Signal Specification2/1
  Signal Specification2/1 -> Bus Assignment/3
  Byte Unpack/3 -> Bus Assignment/5
  Selector1/1 -> Signal Specification1/1
  Signal Specification1/1 -> Bus Assignment/4
